simulink model "motor"  (Simulink 8.6)
settings: Solver=FixedStepDiscrete  StartTime=0.0  StopTime=inf  FixedStep=0.002  RelTol=1e-3
PostLoadFcn:
  | ,try, rti_mdl_postloadfcn(bdroot, 'UpdateModel', 160, 'rti1104'); catch, disp(lasterr); end,
undefined symbols (not defined in the file): DiscIntNeverNeededParam
libraries: simulink x3
(part 1 of 3)
CloseFcn:
  | rtwprivate ssgencode ModelCloseRequest two_pisition
settings Model: Creator=Eason  LastModifiedBy=Administrator
settings DataIOCC: SaveFormat=Structure
settings OptimizationCC: BlockReduction=off  OptimizeBlockIOStorage=off  BufferReuse=off  GlobalBufferReuse=off  ExpressionFolding=off  LocalBlockOutputs=off  InitFltsAndDblsToZero=on  OptimizeModelRefInitCode=on  LifeSpan=Inf
settings DebuggingCC: SaveWithParameterizedLinksMsg=none  SignalResolutionControl=TryResolveAllWithWarning  MultiTaskDSMMsg=warning  MultiTaskCondExecSysMsg=none  FcnCallInpInsideContextMsg=UseLocalSettings
settings HardwareCC: ProdLargestAtomicInteger=Long  ProdLargestAtomicFloat=Double  ProdEndianess=LittleEndian  ProdHWDeviceType=ARM Compatible->ARM Cortex  TargetIntDivRoundTo=Zero  TargetEndianess=BigEndian
settings SFSimCC: SimParseCustomCode=off
settings RTWCC: SystemTargetFile=ert.tlc  TemplateMakefile=ert_default_tmf  Description=Embedded Coder  GenerateReport=on  IncludeHyperlinkInReport=on  LaunchReport=on  GenerateTraceInfo=on  GenerateTraceReport=on  GenerateTraceReportSl=on  GenerateTraceReportSf=on  GenerateTraceReportEml=on
settings CodeAppCC: IgnoreCustomStorageClasses=off  CustomSymbolStrType=$N$R$M  InternalIdentifier=Classic
settings ERTTargetCC: MultiwordLength=2048  GenerateSampleERTMain=on  SupportNonFinite=off  SupportComplex=off  ERTCustomFileTemplate=example_file_process.tlc  ConvertIfToSwitch=off  SuppressUnreachableDefaultCases=off
settings ConfigComp: CovSFcnEnable=off

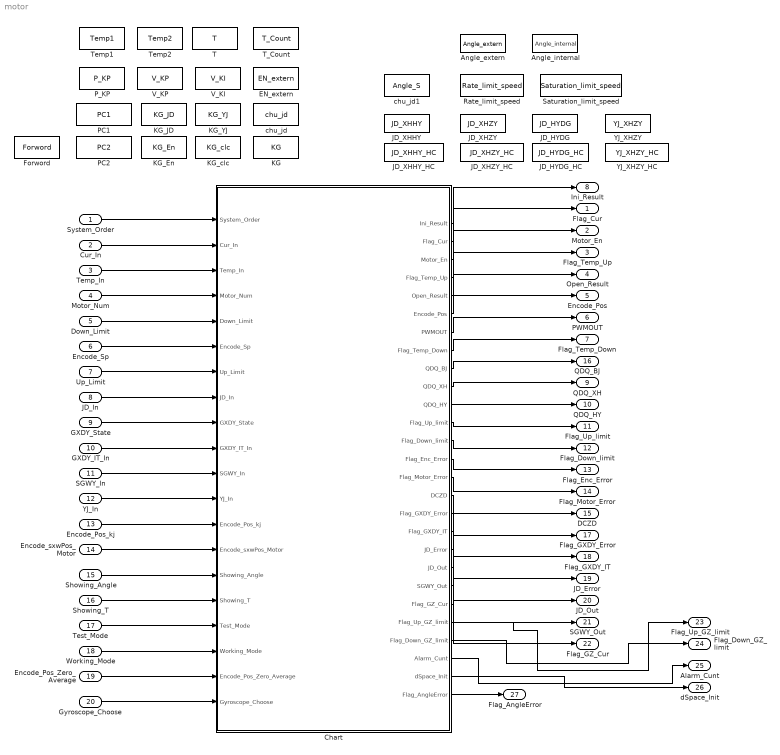
== system motor ==
  System_Order : Inport
  Cur_In : Inport  Port=2  OutDataTypeStr=uint32
  Temp_In : Inport  Port=3  OutDataTypeStr=uint32
  Motor_Num : Inport  Port=4  OutDataTypeStr=uint8
  Down_Limit : Inport  Port=5  OutDataTypeStr=uint8
  Encode_Sp : Inport  Port=6  OutDataTypeStr=int32
  Up_Limit : Inport  Port=7  OutDataTypeStr=uint8
  JD_In : Inport  Port=8  OutDataTypeStr=int32
  GXDY_State : Inport  Port=9  OutDataTypeStr=boolean
  GXDY_IT_In : Inport  Port=10  OutDataTypeStr=uint8
  SGWY_In : Inport  Port=11  OutDataTypeStr=int32
  YJ_In : Inport  Port=12  OutDataTypeStr=int32
  Encode_Pos_kj : Inport  Port=13  OutDataTypeStr=int32
  Encode_sxwPos_Motor : Inport  Port=14  OutDataTypeStr=int32
  Showing_Angle : Inport  Port=15  OutDataTypeStr=int32
  Showing_T : Inport  Port=16  OutDataTypeStr=int32
  Test_Mode : Inport  Port=17  OutDataTypeStr=int32
  Working_Mode : Inport  Port=18  OutDataTypeStr=int32
  Encode_Pos_Zero_Average : Inport  Port=19  OutDataTypeStr=int32
  Gyroscope_Choose : Inport  Port=20  OutDataTypeStr=uint8
  Angle_extern : DataStoreMemory  DataStoreName=Angle_extern  ReadBeforeWriteMsg=warning  WriteAfterWriteMsg=warning  WriteAfterReadMsg=warning  OutDataTypeStr=double
  Angle_internal : DataStoreMemory  DataStoreName=Angle_internal  ReadBeforeWriteMsg=warning  WriteAfterWriteMsg=warning  WriteAfterReadMsg=warning  OutDataTypeStr=double
  Chart : Stateflow chart  TreatAsAtomicUnit=on
  EN_extern : DataStoreMemory  DataStoreName=EN_extern  ReadBeforeWriteMsg=warning  WriteAfterWriteMsg=warning  WriteAfterReadMsg=warning  OutDataTypeStr=uint8
  Forword : DataStoreMemory  DataStoreName=Forword  ReadBeforeWriteMsg=warning  WriteAfterWriteMsg=warning  WriteAfterReadMsg=warning  InitialValue=1  OutDataTypeStr=uint8
  JD_HYDG : DataStoreMemory  DataStoreName=JD_HYDG  ReadBeforeWriteMsg=warning  WriteAfterWriteMsg=warning  WriteAfterReadMsg=warning  OutDataTypeStr=int32
  JD_HYDG_HC : DataStoreMemory  DataStoreName=JD_HYDG_HC  ReadBeforeWriteMsg=warning  WriteAfterWriteMsg=warning  WriteAfterReadMsg=warning  OutDataTypeStr=int32
  JD_XHHY : DataStoreMemory  DataStoreName=JD_XHHY  ReadBeforeWriteMsg=warning  WriteAfterWriteMsg=warning  WriteAfterReadMsg=warning  OutDataTypeStr=int32
  JD_XHHY_HC : DataStoreMemory  DataStoreName=JD_XHHY_HC  ReadBeforeWriteMsg=warning  WriteAfterWriteMsg=warning  WriteAfterReadMsg=warning  OutDataTypeStr=int32
  JD_XHZY : DataStoreMemory  DataStoreName=JD_XHZY  ReadBeforeWriteMsg=warning  WriteAfterWriteMsg=warning  WriteAfterReadMsg=warning  OutDataTypeStr=int32
  JD_XHZY_HC : DataStoreMemory  DataStoreName=JD_XHZY_HC  ReadBeforeWriteMsg=warning  WriteAfterWriteMsg=warning  WriteAfterReadMsg=warning  OutDataTypeStr=int32
  KG : DataStoreMemory  DataStoreName=KG  ReadBeforeWriteMsg=warning  WriteAfterWriteMsg=warning  WriteAfterReadMsg=warning  OutDataTypeStr=uint8
  KG_En : DataStoreMemory  DataStoreName=KG_En  ReadBeforeWriteMsg=warning  WriteAfterWriteMsg=warning  WriteAfterReadMsg=warning  OutDataTypeStr=uint8
  KG_JD : DataStoreMemory  DataStoreName=KG_JD  ReadBeforeWriteMsg=warning  WriteAfterWriteMsg=warning  WriteAfterReadMsg=warning  OutDataTypeStr=uint8
  KG_YJ : DataStoreMemory  DataStoreName=KG_YJ  ReadBeforeWriteMsg=warning  WriteAfterWriteMsg=warning  WriteAfterReadMsg=warning  OutDataTypeStr=uint8
  KG_clc : DataStoreMemory  DataStoreName=KG_clc  ReadBeforeWriteMsg=warning  WriteAfterWriteMsg=warning  WriteAfterReadMsg=warning  OutDataTypeStr=uint8
  PC1 : DataStoreMemory  DataStoreName=PC1  ReadBeforeWriteMsg=warning  WriteAfterWriteMsg=warning  WriteAfterReadMsg=warning  OutDataTypeStr=boolean
  PC2 : DataStoreMemory  DataStoreName=PC2  ReadBeforeWriteMsg=warning  WriteAfterWriteMsg=warning  WriteAfterReadMsg=warning  OutDataTypeStr=boolean
  P_KP : DataStoreMemory  DataStoreName=P_KP  ReadBeforeWriteMsg=warning  WriteAfterWriteMsg=warning  WriteAfterReadMsg=warning  InitialValue=330  OutDataTypeStr=double
  Rate_limit_speed : DataStoreMemory  DataStoreName=Rate_limit_speed  ReadBeforeWriteMsg=warning  WriteAfterWriteMsg=warning  WriteAfterReadMsg=warning  InitialValue=50000  OutDataTypeStr=double
  Saturation_limit_speed : DataStoreMemory  DataStoreName=Saturation_limit_speed  ReadBeforeWriteMsg=warning  WriteAfterWriteMsg=warning  WriteAfterReadMsg=warning  InitialValue=16000  OutDataTypeStr=double
  T : DataStoreMemory  DataStoreName=T  ReadBeforeWriteMsg=warning  WriteAfterWriteMsg=warning  WriteAfterReadMsg=warning  OutDataTypeStr=double
  T_Count : DataStoreMemory  DataStoreName=T_Count  ReadBeforeWriteMsg=warning  WriteAfterWriteMsg=warning  WriteAfterReadMsg=warning  OutDataTypeStr=double
  Temp1 : DataStoreMemory  DataStoreName=Temp1  ReadBeforeWriteMsg=warning  WriteAfterWriteMsg=warning  WriteAfterReadMsg=warning  OutDataTypeStr=double
  Temp2 : DataStoreMemory  DataStoreName=Temp2  ReadBeforeWriteMsg=warning  WriteAfterWriteMsg=warning  WriteAfterReadMsg=warning  OutDataTypeStr=double
  V_KI : DataStoreMemory  DataStoreName=V_KI  ReadBeforeWriteMsg=warning  WriteAfterWriteMsg=warning  WriteAfterReadMsg=warning  InitialValue=10  OutDataTypeStr=double
  V_KP : DataStoreMemory  DataStoreName=V_KP  ReadBeforeWriteMsg=warning  WriteAfterWriteMsg=warning  WriteAfterReadMsg=warning  InitialValue=1  OutDataTypeStr=double
  YJ_XHZY : DataStoreMemory  DataStoreName=YJ_XHZY  ReadBeforeWriteMsg=warning  WriteAfterWriteMsg=warning  WriteAfterReadMsg=warning  OutDataTypeStr=int32
  YJ_XHZY_HC : DataStoreMemory  DataStoreName=YJ_XHZY_HC  ReadBeforeWriteMsg=warning  WriteAfterWriteMsg=warning  WriteAfterReadMsg=warning  OutDataTypeStr=int32
  chu_jd : DataStoreMemory  DataStoreName=chu_jd  ReadBeforeWriteMsg=warning  WriteAfterWriteMsg=warning  WriteAfterReadMsg=warning  OutDataTypeStr=double
  chu_jd1 : DataStoreMemory  DataStoreName=Angle_S  ReadBeforeWriteMsg=warning  WriteAfterWriteMsg=warning  WriteAfterReadMsg=warning  OutDataTypeStr=double
  Flag_Cur : Outport  OutDataTypeStr=uint8
  Motor_En : Outport  Port=2  OutDataTypeStr=boolean
  Flag_Temp_Up : Outport  Port=3  OutDataTypeStr=uint8
  Open_Result : Outport  Port=4  OutDataTypeStr=uint8
  Encode_Pos : Outport  Port=5  OutDataTypeStr=int32
  PWMOUT : Outport  Port=6  OutDataTypeStr=uint16
  Flag_Temp_Down : Outport  Port=7  OutDataTypeStr=uint8
  Ini_Result : Outport  Port=8  OutDataTypeStr=uint8
  QDQ_XH : Outport  Port=9  OutDataTypeStr=boolean
  QDQ_HY : Outport  Port=10  OutDataTypeStr=boolean
  Flag_Up_limit : Outport  Port=11  OutDataTypeStr=uint8
  Flag_Down_limit : Outport  Port=12  OutDataTypeStr=uint8
  Flag_Enc_Error : Outport  Port=13  OutDataTypeStr=uint8
  Flag_Motor_Error : Outport  Port=14  OutDataTypeStr=uint8
  DCZD : Outport  Port=15  OutDataTypeStr=boolean
  QDQ_BJ : Outport  Port=16  OutDataTypeStr=uint8
  Flag_GXDY_Error : Outport  Port=17  OutDataTypeStr=uint8
  Flag_GXDY_IT : Outport  Port=18  OutDataTypeStr=uint8
  JD_Error : Outport  Port=19  OutDataTypeStr=int32
  JD_Out : Outport  Port=20  OutDataTypeStr=int32
  SGWY_Out : Outport  Port=21  OutDataTypeStr=int32
  Flag_GZ_Cur : Outport  Port=22  OutDataTypeStr=uint8
  Flag_Up_GZ_limit : Outport  Port=23  OutDataTypeStr=uint8
  Flag_Down_GZ_limit : Outport  Port=24  OutDataTypeStr=uint8
  Alarm_Cunt : Outport  Port=25  OutDataTypeStr=uint8
  dSpace_Init : Outport  Port=26  OutDataTypeStr=uint8
  Flag_AngleError : Outport  Port=27  OutDataTypeStr=uint8
  wires:
  Chart/2(Flag_Cur) -> Flag_Cur/1
  Chart/3(Motor_En) -> Motor_En/1
  Temp_In/1 -> Chart/3(Temp_In)
  Chart/4(Flag_Temp_Up) -> Flag_Temp_Up/1
  Chart/5(Open_Result) -> Open_Result/1
  Motor_Num/1 -> Chart/4(Motor_Num)
  Chart/6(Encode_Pos) -> Encode_Pos/1
  Chart/7(PWMOUT) -> PWMOUT/1
  Chart/8(Flag_Temp_Down) -> Flag_Temp_Down/1
  Chart/1(Ini_Result) -> Ini_Result/1
  Chart/10(QDQ_XH) -> QDQ_XH/1
  Chart/11(QDQ_HY) -> QDQ_HY/1
  Cur_In/1 -> Chart/2(Cur_In)
  System_Order/1 -> Chart/1(System_Order)
  Chart/12(Flag_Up_limit) -> Flag_Up_limit/1
  Chart/13(Flag_Down_limit) -> Flag_Down_limit/1
  Chart/14(Flag_Enc_Error) -> Flag_Enc_Error/1
  Chart/15(Flag_Motor_Error) -> Flag_Motor_Error/1
  Chart/16(DCZD) -> DCZD/1
  Down_Limit/1 -> Chart/5(Down_Limit)
  Encode_Sp/1 -> Chart/6(Encode_Sp)
  Chart/9(QDQ_BJ) -> QDQ_BJ/1
  JD_In/1 -> Chart/8(JD_In)
  Chart/17(Flag_GXDY_Error) -> Flag_GXDY_Error/1
  GXDY_State/1 -> Chart/9(GXDY_State)
  GXDY_IT_In/1 -> Chart/10(GXDY_IT_In)
  Chart/18(Flag_GXDY_IT) -> Flag_GXDY_IT/1
  SGWY_In/1 -> Chart/11(SGWY_In)
  YJ_In/1 -> Chart/12(YJ_In)
  Chart/19(JD_Error) -> JD_Error/1
  Chart/20(JD_Out) -> JD_Out/1
  Chart/21(SGWY_Out) -> SGWY_Out/1
  Chart/22(Flag_GZ_Cur) -> Flag_GZ_Cur/1
  Chart/23(Flag_Up_GZ_limit) -> Flag_Up_GZ_limit/1
  Chart/24(Flag_Down_GZ_limit) -> Flag_Down_GZ_limit/1
  Chart/25(Alarm_Cunt) -> Alarm_Cunt/1
  Encode_Pos_kj/1 -> Chart/13(Encode_Pos_kj)
  Encode_sxwPos_Motor/1 -> Chart/14(Encode_sxwPos_Motor)
  Up_Limit/1 -> Chart/7(Up_Limit)
  Showing_Angle/1 -> Chart/15(Showing_Angle)
  Showing_T/1 -> Chart/16(Showing_T)
  Test_Mode/1 -> Chart/17(Test_Mode)
  Working_Mode/1 -> Chart/18(Working_Mode)
  Encode_Pos_Zero_Average/1 -> Chart/19(Encode_Pos_Zero_Average)
  Gyroscope_Choose/1 -> Chart/20(Gyroscope_Choose)
  Chart/26(dSpace_Init) -> dSpace_Init/1
  Chart/27(Flag_AngleError) -> Flag_AngleError/1

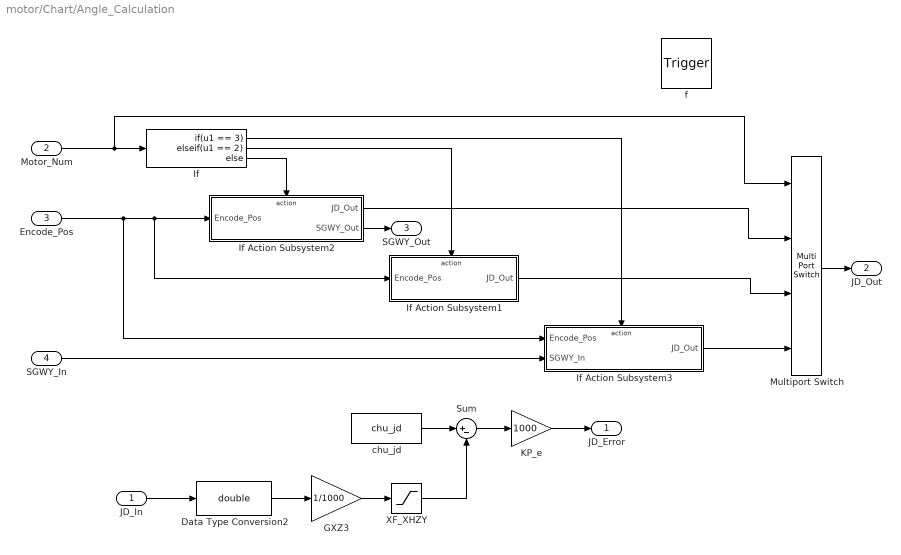
== system motor/Chart/Angle_Calculation ==
  JD_In : Inport  OutDataTypeStr=int32  PortDimensions=1
  Motor_Num : Inport  Port=2  OutDataTypeStr=uint8  PortDimensions=1
  Encode_Pos : Inport  Port=3  OutDataTypeStr=uint8  PortDimensions=1
  SGWY_In : Inport  Port=4  OutDataTypeStr=uint8  PortDimensions=1
  f : TriggerPort  TriggerType=function-call
      settings: CopyFcn=Stateflow.SLINSF.SimulinkMan.removeBlockPreDeleteFcn  PreDeleteFcn=Stateflow.SLINSF.SimulinkMan.unsafePredeleteFcn
  Data Type Conversion2 : DataTypeConversion  OutDataTypeStr=double
  GXZ3 : Gain  Gain=1/1000
  If : If  IfExpression=u1 == 3  ElseIfExpressions=u1 == 2
  If Action Subsystem1 : Subsystem  TreatAsAtomicUnit=on
  If Action Subsystem2 : Subsystem  TreatAsAtomicUnit=on
  If Action Subsystem3 : Subsystem  TreatAsAtomicUnit=on
  KP_e : Gain  Gain=1000
  Multiport Switch : MultiPortSwitch
  Sum : Sum  Inputs=|+-
  XF_XHZY : Saturate  UpperLimit=15  LowerLimit=-15
  chu_jd : DataStoreRead  DataStoreName=chu_jd
  JD_Error : Outport
  JD_Out : Outport  Port=2
  SGWY_Out : Outport  Port=3
  wires:
  GXZ3/1 -> XF_XHZY/1
  XF_XHZY/1 -> Sum/2
  Data Type Conversion2/1 -> GXZ3/1
  If/1 -> If Action Subsystem3/Action
  If/2 -> If Action Subsystem1/Action
  If/3 -> If Action Subsystem2/Action
  Motor_Num/1 -> Multiport Switch/1, If/1
  JD_In/1 -> Data Type Conversion2/1
  Sum/1 -> KP_e/1
  KP_e/1 -> JD_Error/1
  chu_jd/1 -> Sum/1
  Encode_Pos/1 -> If Action Subsystem3/1(Encode_Pos), If Action Subsystem1/1(Encode_Pos), If Action Subsystem2/1(Encode_Pos)
  SGWY_In/1 -> If Action Subsystem3/2(SGWY_In)
  If Action Subsystem2/2(SGWY_Out) -> SGWY_Out/1
  If Action Subsystem3/1(JD_Out) -> Multiport Switch/4
  If Action Subsystem1/1(JD_Out) -> Multiport Switch/3
  If Action Subsystem2/1(JD_Out) -> Multiport Switch/2
  Multiport Switch/1 -> JD_Out/1

== system motor/Chart/Angle_Calculation_HY ==
  Encode_Pos : Inport  OutDataTypeStr=int32  PortDimensions=1
  f : TriggerPort  TriggerType=function-call
      settings: CopyFcn=Stateflow.SLINSF.SimulinkMan.removeBlockPreDeleteFcn  PreDeleteFcn=Stateflow.SLINSF.SimulinkMan.unsafePredeleteFcn
  Data Type Conversion1 : DataTypeConversion  OutDataTypeStr=double
  GHDG5 : Gain  Gain=360/65536
  fs_plat : Subsystem
  Angle_Calculation : Outport
  wires:
  Encode_Pos/1 -> Data Type Conversion1/1
  Data Type Conversion1/1 -> GHDG5/1
  GHDG5/1 -> fs_plat/1(In1)
  fs_plat/1(Out1) -> Angle_Calculation/1

== system motor/Chart/Angle_Calculation_XH ==
  Encode_Pos : Inport  OutDataTypeStr=int32  PortDimensions=1
  f : TriggerPort  TriggerType=function-call
      settings: CopyFcn=Stateflow.SLINSF.SimulinkMan.removeBlockPreDeleteFcn  PreDeleteFcn=Stateflow.SLINSF.SimulinkMan.unsafePredeleteFcn
  Data Type Conversion2 : DataTypeConversion  OutDataTypeStr=double
  GXZ1 : Gain  Gain=1/322
  GXZ6 : Gain  Gain=360/65536
  Angle_Calculation : Outport
  wires:
  Encode_Pos/1 -> Data Type Conversion2/1
  GXZ6/1 -> GXZ1/1
  Data Type Conversion2/1 -> GXZ6/1
  GXZ1/1 -> Angle_Calculation/1

== system motor/Chart/BJ ==
  x : Inport  OutDataTypeStr=uint8
  y : Inport  Port=2
  f : TriggerPort  TriggerType=function-call
      settings: CopyFcn=Stateflow.SLINSF.SimulinkMan.removeBlockPreDeleteFcn  PreDeleteFcn=Stateflow.SLINSF.SimulinkMan.unsafePredeleteFcn
  Data Store Read : DataStoreRead  DataStoreName=PC2
  Data Store Read1 : DataStoreRead  DataStoreName=PC1
  If Action Subsystem : Subsystem  TreatAsAtomicUnit=on
  If Action Subsystem1 : Subsystem  TreatAsAtomicUnit=on
  If Action Subsystem2 : Subsystem  TreatAsAtomicUnit=on
  Switch Case : SwitchCase  CaseConditions={1 2 3}  ShowDefaultCase=off
  Out1 : Outport  OutDataTypeStr=boolean
  Out2 : Outport  Port=2  OutDataTypeStr=boolean
  wires:
  Switch Case/1 -> If Action Subsystem/Action
  Switch Case/2 -> If Action Subsystem1/Action
  Switch Case/3 -> If Action Subsystem2/Action
  y/1 -> If Action Subsystem2/1(In1), If Action Subsystem1/1(In1), If Action Subsystem/1(In1)
  x/1 -> Switch Case/1
  Data Store Read1/1 -> Out1/1
  Data Store Read/1 -> Out2/1

== system motor/Chart/COM_Error ==
  In : Inport
  f : TriggerPort  TriggerType=function-call
      settings: CopyFcn=Stateflow.SLINSF.SimulinkMan.removeBlockPreDeleteFcn  PreDeleteFcn=Stateflow.SLINSF.SimulinkMan.unsafePredeleteFcn
  Abs : Abs
  Add : Sum  Inputs=+-
  Unit Delay : UnitDelay  SampleTime=-1
  Out : Outport
  wires:
  In/1 -> Unit Delay/1, Add/1
  Unit Delay/1 -> Add/2
  Add/1 -> Abs/1
  Abs/1 -> Out/1

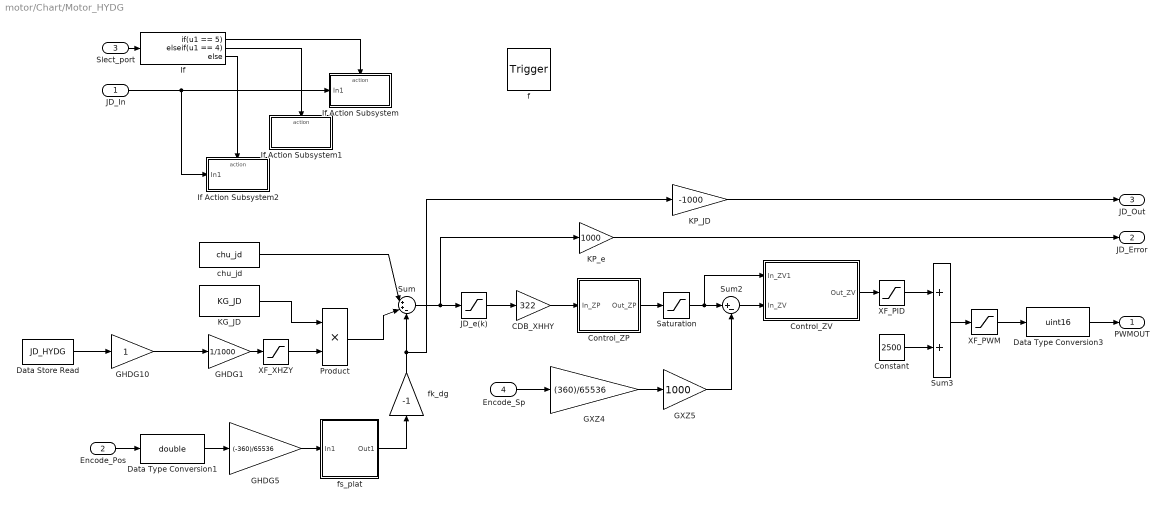
== system motor/Chart/Motor_HYDG ==
  JD_In : Inport  OutDataTypeStr=int32  PortDimensions=1
  Encode_Pos : Inport  Port=2  OutDataTypeStr=int32  PortDimensions=1
  Slect_port : Inport  Port=3  OutDataTypeStr=uint8  PortDimensions=1
  Encode_Sp : Inport  Port=4  OutDataTypeStr=int32  PortDimensions=1
  f : TriggerPort  TriggerType=function-call
      settings: CopyFcn=Stateflow.SLINSF.SimulinkMan.removeBlockPreDeleteFcn  PreDeleteFcn=Stateflow.SLINSF.SimulinkMan.unsafePredeleteFcn
  CDB_XHHY : Gain  Gain=322
  Constant : Constant  Value=2500
  Control_ZP : Subsystem
  Control_ZV : Subsystem
  Data Store Read : DataStoreRead  DataStoreName=JD_HYDG
  Data Type Conversion1 : DataTypeConversion  OutDataTypeStr=double
  Data Type Conversion3 : DataTypeConversion  OutDataTypeStr=uint16
  GHDG1 : Gain  Gain=1/1000
  GHDG10 : Gain
  GHDG5 : Gain  Gain=(-360)/65536
  GXZ4 : Gain  Gain=(360)/65536
  GXZ5 : Gain  Gain=1000
  If : If  IfExpression=u1 == 5  ElseIfExpressions=u1 == 4
  If Action Subsystem : Subsystem  TreatAsAtomicUnit=on
  If Action Subsystem1 : Subsystem  TreatAsAtomicUnit=on
  If Action Subsystem2 : Subsystem  TreatAsAtomicUnit=on
  JD_e(k) : Saturate  UpperLimit=15  LowerLimit=-15
  KG_JD : DataStoreRead  DataStoreName=KG_JD
  KP_JD : Gain  Gain=-1000
  KP_e : Gain  Gain=1000
  Product : Product  OutDataTypeStr=double
  Saturation : Saturate  UpperLimit=8000  LowerLimit=-8000
  Sum : Sum  Inputs=|++-
  Sum2 : Sum  Inputs=|+-
  Sum3 : Sum
  XF_PID : Saturate  UpperLimit=2500  LowerLimit=-2500
  XF_PWM : Saturate  UpperLimit=4000  LowerLimit=1000
  XF_XHZY : Saturate  UpperLimit=15  LowerLimit=-15
  chu_jd : DataStoreRead  DataStoreName=chu_jd
  fk_dg : Gain  Gain=-1
  fs_plat : Subsystem
  PWMOUT : Outport
  JD_Error : Outport  Port=2
  JD_Out : Outport  Port=3
  wires:
  Product/1 -> Sum/2
  Control_ZV/1(Out_ZV) -> XF_PID/1
  XF_PID/1 -> Sum3/1
  Constant/1 -> Sum3/2
  Sum3/1 -> XF_PWM/1
  XF_PWM/1 -> Data Type Conversion3/1
  GHDG10/1 -> GHDG1/1
  GHDG1/1 -> XF_XHZY/1
  KG_JD/1 -> Product/1
  Encode_Pos/1 -> Data Type Conversion1/1
  Data Type Conversion3/1 -> PWMOUT/1
  KP_JD/1 -> JD_Out/1
  KP_e/1 -> JD_Error/1
  Data Store Read/1 -> GHDG10/1
  JD_In/1 -> If Action Subsystem2/1(In1), If Action Subsystem/1(In1)
  If/1 -> If Action Subsystem/Action
  If/2 -> If Action Subsystem1/Action
  If/3 -> If Action Subsystem2/Action
  Slect_port/1 -> If/1
  Data Type Conversion1/1 -> GHDG5/1
  GXZ4/1 -> GXZ5/1
  Encode_Sp/1 -> GXZ4/1
  XF_XHZY/1 -> Product/2
  CDB_XHHY/1 -> Control_ZP/1(In_ZP)
  Control_ZP/1(Out_ZP) -> Saturation/1
  Sum2/1 -> Control_ZV/2(In_ZV)
  Sum/1 -> KP_e/1, JD_e(k)/1
  Saturation/1 -> Sum2/1, Control_ZV/1(In_ZV1)
  JD_e(k)/1 -> CDB_XHHY/1
  GXZ5/1 -> Sum2/2
  fk_dg/1 -> KP_JD/1, Sum/3
  chu_jd/1 -> Sum/1
  GHDG5/1 -> fs_plat/1(In1)
  fs_plat/1(Out1) -> fk_dg/1

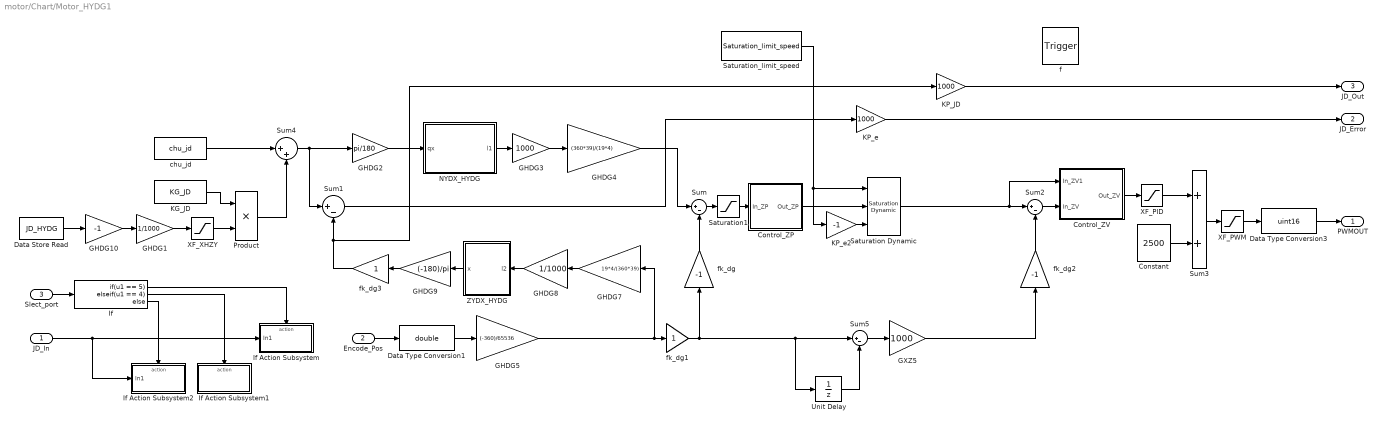
== system motor/Chart/Motor_HYDG1 ==
  JD_In : Inport  OutDataTypeStr=int32  PortDimensions=1
  Encode_Pos : Inport  Port=2  OutDataTypeStr=int32  PortDimensions=1
  Slect_port : Inport  Port=3  OutDataTypeStr=uint8  PortDimensions=1
  f : TriggerPort  TriggerType=function-call
      settings: CopyFcn=Stateflow.SLINSF.SimulinkMan.removeBlockPreDeleteFcn  PreDeleteFcn=Stateflow.SLINSF.SimulinkMan.unsafePredeleteFcn
  Constant : Constant  Value=2500
  Control_ZP : Subsystem
  Control_ZV : Subsystem
  Data Store Read : DataStoreRead  DataStoreName=JD_HYDG
  Data Type Conversion1 : DataTypeConversion  OutDataTypeStr=double
  Data Type Conversion3 : DataTypeConversion  OutDataTypeStr=uint16
  GHDG1 : Gain  Gain=1/1000
  GHDG10 : Gain  Gain=-1
  GHDG2 : Gain  Gain=pi/180
  GHDG3 : Gain  Gain=1000
  GHDG4 : Gain  Gain=(360*39)/(19*4)
  GHDG5 : Gain  Gain=(-360)/65536
  GHDG7 : Gain  Gain=19*4/(360*39)
  GHDG8 : Gain  Gain=1/1000
  GHDG9 : Gain  Gain=(-180)/pi
  GXZ5 : Gain  Gain=1000
  If : If  IfExpression=u1 == 5  ElseIfExpressions=u1 == 4
  If Action Subsystem : Subsystem  TreatAsAtomicUnit=on
  If Action Subsystem1 : Subsystem  TreatAsAtomicUnit=on
  If Action Subsystem2 : Subsystem  TreatAsAtomicUnit=on
  KG_JD : DataStoreRead  DataStoreName=KG_JD
  KP_JD : Gain  Gain=1000
  KP_e : Gain  Gain=1000
  KP_e2 : Gain  Gain=-1
  NYDX_HYDG : Subsystem
  Product : Product  OutDataTypeStr=double
  Saturation Dynamic : simulink/Discontinuities/Saturation Dynamic  OutMin=[]  OutMax=[]  OutDataTypeStr=Inherit: Same as second input  OutDataType=fixdt(1, 16)  OutScaling=2^-10  DoSatur=off
  Saturation1 : Saturate  UpperLimit=200  LowerLimit=-200
  Saturation_limit_speed : DataStoreRead  DataStoreName=Saturation_limit_speed
  Sum{,1..2,5} (4 alike) : Sum  Inputs=|+-
  Sum3 : Sum
  Sum4 : Sum  Inputs=|++
  Unit Delay : UnitDelay  SampleTime=-1
  XF_PID : Saturate  UpperLimit=2500  LowerLimit=-2500
  XF_PWM : Saturate  UpperLimit=4900  LowerLimit=100
  XF_XHZY : Saturate  UpperLimit=20  LowerLimit=-20
  ZYDX_HYDG : Subsystem
  chu_jd : DataStoreRead  DataStoreName=chu_jd
  fk_dg : Gain  Gain=-1
  fk_dg1 : Gain
  fk_dg2 : Gain  Gain=-1
  fk_dg3 : Gain
  PWMOUT : Outport
  JD_Error : Outport  Port=2
  JD_Out : Outport  Port=3
  wires:
  GHDG4/1 -> Sum/1
  Control_ZV/1(Out_ZV) -> XF_PID/1
  XF_PID/1 -> Sum3/1
  Constant/1 -> Sum3/2
  Sum3/1 -> XF_PWM/1
  XF_PWM/1 -> Data Type Conversion3/1
  GHDG10/1 -> GHDG1/1
  GHDG1/1 -> XF_XHZY/1
  KG_JD/1 -> Product/1
  Encode_Pos/1 -> Data Type Conversion1/1
  Data Type Conversion3/1 -> PWMOUT/1
  KP_JD/1 -> JD_Out/1
  KP_e/1 -> JD_Error/1
  Data Store Read/1 -> GHDG10/1
  JD_In/1 -> If Action Subsystem2/1(In1), If Action Subsystem/1(In1)
  If/1 -> If Action Subsystem/Action
  If/2 -> If Action Subsystem1/Action
  If/3 -> If Action Subsystem2/Action
  Slect_port/1 -> If/1
  Data Type Conversion1/1 -> GHDG5/1
  XF_XHZY/1 -> Product/2
  Sum/1 -> Saturation1/1
  Control_ZP/1(Out_ZP) -> Saturation Dynamic/2
  Sum2/1 -> Control_ZV/2(In_ZV)
  GXZ5/1 -> fk_dg2/1
  fk_dg/1 -> Sum/2
  GHDG2/1 -> NYDX_HYDG/1(qx)
  NYDX_HYDG/1(l1) -> GHDG3/1
  GHDG3/1 -> GHDG4/1
  Product/1 -> Sum4/2
  GHDG5/1 -> fk_dg1/1, GHDG7/1
  GHDG7/1 -> GHDG8/1
  GHDG8/1 -> ZYDX_HYDG/1(l2)
  ZYDX_HYDG/1(x) -> GHDG9/1
  Sum1/1 -> KP_e/1
  GHDG9/1 -> fk_dg3/1
  fk_dg3/1 -> Sum1/2, KP_JD/1
  Sum5/1 -> GXZ5/1
  Sum4/1 -> Sum1/1, GHDG2/1
  chu_jd/1 -> Sum4/1
  Unit Delay/1 -> Sum5/2
  fk_dg1/1 -> Unit Delay/1, Sum5/1, fk_dg/1
  fk_dg2/1 -> Sum2/2
  Saturation1/1 -> Control_ZP/1(In_ZP)
  Saturation Dynamic/1 -> Sum2/1, Control_ZV/1(In_ZV1)
  Saturation_limit_speed/1 -> KP_e2/1, Saturation Dynamic/1
  KP_e2/1 -> Saturation Dynamic/3

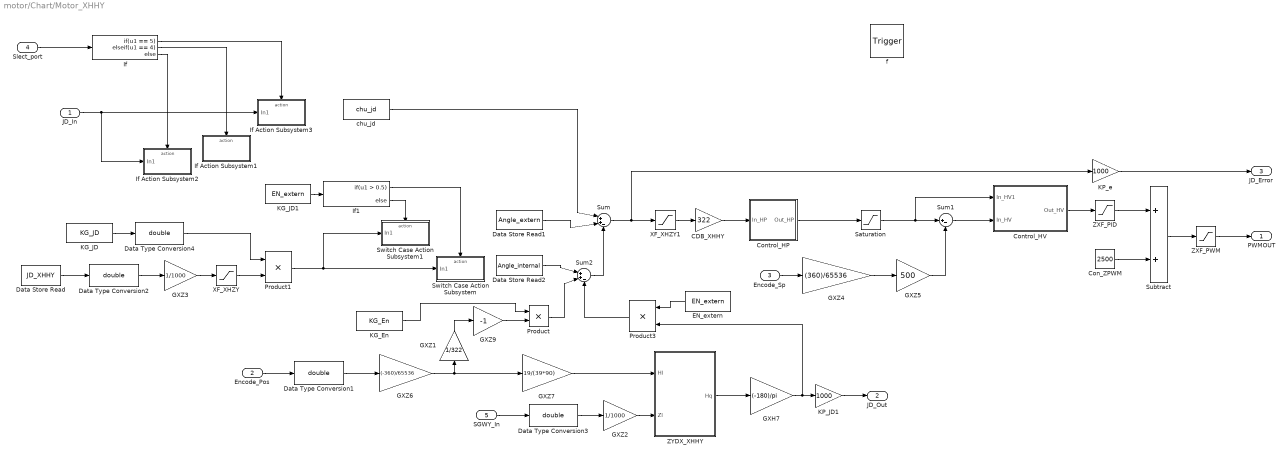
== system motor/Chart/Motor_XHHY ==
  JD_In : Inport  OutDataTypeStr=int32  PortDimensions=1
  Encode_Pos : Inport  Port=2  OutDataTypeStr=int32  PortDimensions=1
  Encode_Sp : Inport  Port=3  OutDataTypeStr=int32  PortDimensions=1
  Slect_port : Inport  Port=4  OutDataTypeStr=uint8  PortDimensions=1
  SGWY_In : Inport  Port=5  OutDataTypeStr=int32  PortDimensions=1
  f : TriggerPort  TriggerType=function-call
      settings: CopyFcn=Stateflow.SLINSF.SimulinkMan.removeBlockPreDeleteFcn  PreDeleteFcn=Stateflow.SLINSF.SimulinkMan.unsafePredeleteFcn
  CDB_XHHY : Gain  Gain=322
  Con_ZPWM : Constant  Value=2500
  Control_HP : Subsystem
  Control_HV : Subsystem
  Data Store Read : DataStoreRead  DataStoreName=JD_XHHY
  Data Store Read1 : DataStoreRead  DataStoreName=Angle_extern
  Data Store Read2 : DataStoreRead  DataStoreName=Angle_internal
  Data Type Conversion{1..4} (4 alike) : DataTypeConversion  OutDataTypeStr=double
  EN_extern : DataStoreRead  DataStoreName=EN_extern
  GXH7 : Gain  Gain=(-180)/pi
  GXZ1 : Gain  Gain=1/322
  GXZ2 : Gain  Gain=1/1000
  GXZ3 : Gain  Gain=1/1000
  GXZ4 : Gain  Gain=(360)/65536
  GXZ5 : Gain  Gain=500
  GXZ6 : Gain  Gain=(-360)/65536
  GXZ7 : Gain  Gain=19/(39*90)
  GXZ9 : Gain  Gain=-1
  If : If  IfExpression=u1 == 5  ElseIfExpressions=u1 == 4
  If Action Subsystem1 : Subsystem  TreatAsAtomicUnit=on
  If Action Subsystem2 : Subsystem  TreatAsAtomicUnit=on
  If Action Subsystem3 : Subsystem  TreatAsAtomicUnit=on
  If1 : If  IfExpression=u1 > 0.5
  KG_En : DataStoreRead  DataStoreName=KG_En
  KG_JD : DataStoreRead  DataStoreName=KG_JD
  KG_JD1 : DataStoreRead  DataStoreName=EN_extern
  KP_JD1 : Gain  Gain=1000
  KP_e : Gain  Gain=1000
  Product : Product
  Product1 : Product
  Product3 : Product
  Saturation : Saturate  UpperLimit=6600  LowerLimit=-6600
  Subtract : Sum
  Sum : Sum  Inputs=|++-
  Sum1 : Sum  Inputs=|+-
  Sum2 : Sum  Inputs=|++-
  Switch Case Action Subsystem : Subsystem  TreatAsAtomicUnit=on
  Switch Case Action Subsystem1 : Subsystem  TreatAsAtomicUnit=on
  XF_XHZY : Saturate  UpperLimit=15  LowerLimit=-15
  XF_XHZY1 : Saturate  UpperLimit=15  LowerLimit=-15
  ZXF_PID : Saturate  UpperLimit=2500  LowerLimit=-2500
  ZXF_PWM : Saturate  UpperLimit=4800  LowerLimit=200
  ZYDX_XHHY : Subsystem
  chu_jd : DataStoreRead  DataStoreName=chu_jd
  PWMOUT : Outport
  JD_Out : Outport  Port=2
  JD_Error : Outport  Port=3
  wires:
  CDB_XHHY/1 -> Control_HP/1(In_HP)
  Control_HP/1(Out_HP) -> Saturation/1
  Sum1/1 -> Control_HV/2(In_HV)
  Control_HV/1(Out_HV) -> ZXF_PID/1
  ZXF_PID/1 -> Subtract/1
  Con_ZPWM/1 -> Subtract/2
  Subtract/1 -> ZXF_PWM/1
  ZXF_PWM/1 -> PWMOUT/1
  GXZ5/1 -> Sum1/2
  Encode_Sp/1 -> GXZ4/1
  GXZ4/1 -> GXZ5/1
  Encode_Pos/1 -> Data Type Conversion1/1
  GXZ6/1 -> GXZ7/1, GXZ1/1
  GXZ3/1 -> XF_XHZY/1
  Saturation/1 -> Control_HV/1(In_HV1), Sum1/1
  GXZ1/1 -> GXZ9/1
  Product/1 -> Sum2/2
  KG_En/1 -> Product/1
  Data Type Conversion1/1 -> GXZ6/1
  Data Type Conversion2/1 -> GXZ3/1
  JD_In/1 -> If Action Subsystem3/1(In1), If Action Subsystem2/1(In1)
  If/1 -> If Action Subsystem3/Action
  If/2 -> If Action Subsystem1/Action
  If/3 -> If Action Subsystem2/Action
  Slect_port/1 -> If/1
  Data Store Read/1 -> Data Type Conversion2/1
  Sum/1 -> XF_XHZY1/1, KP_e/1
  GXZ9/1 -> Product/2
  KP_e/1 -> JD_Error/1
  ZYDX_XHHY/1(Hq) -> GXH7/1
  GXZ7/1 -> ZYDX_XHHY/1(Hl)
  SGWY_In/1 -> Data Type Conversion3/1
  GXZ2/1 -> ZYDX_XHHY/2(Zl)
  KP_JD1/1 -> JD_Out/1
  Data Type Conversion3/1 -> GXZ2/1
  XF_XHZY1/1 -> CDB_XHHY/1
  XF_XHZY/1 -> Product1/2
  KG_JD/1 -> Data Type Conversion4/1
  Data Type Conversion4/1 -> Product1/1
  chu_jd/1 -> Sum/1
  GXH7/1 -> Product3/2, KP_JD1/1
  Product3/1 -> Sum2/3
  EN_extern/1 -> Product3/1
  Sum2/1 -> Sum/3
  KG_JD1/1 -> If1/1
  If1/1 -> Switch Case Action Subsystem/Action
  Data Store Read1/1 -> Sum/2
  Data Store Read2/1 -> Sum2/1
  Product1/1 -> Switch Case Action Subsystem1/1(In1), Switch Case Action Subsystem/1(In1)
  If1/2 -> Switch Case Action Subsystem1/Action

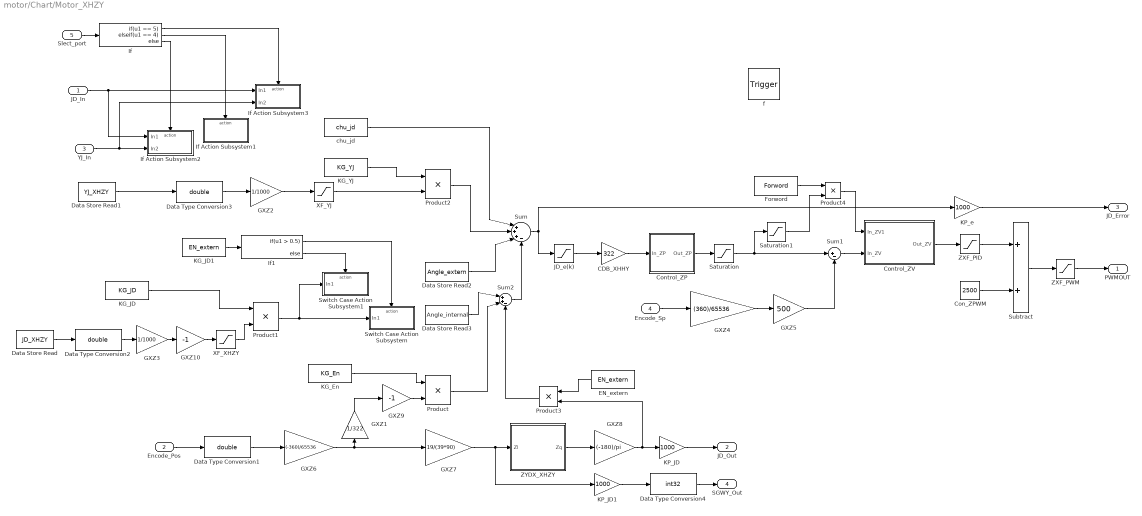
== system motor/Chart/Motor_XHZY ==
  JD_In : Inport  OutDataTypeStr=int32  PortDimensions=1
  Encode_Pos : Inport  Port=2  OutDataTypeStr=int32  PortDimensions=1
  YJ_In : Inport  Port=3  OutDataTypeStr=int32  PortDimensions=1
  Encode_Sp : Inport  Port=4  OutDataTypeStr=int32  PortDimensions=1
  Slect_port : Inport  Port=5  OutDataTypeStr=uint8  PortDimensions=1
  f : TriggerPort  TriggerType=function-call
      settings: CopyFcn=Stateflow.SLINSF.SimulinkMan.removeBlockPreDeleteFcn  PreDeleteFcn=Stateflow.SLINSF.SimulinkMan.unsafePredeleteFcn
  CDB_XHHY : Gain  Gain=322
  Con_ZPWM : Constant  Value=2500
  Control_ZP : Subsystem
  Control_ZV : Subsystem
  Data Store Read : DataStoreRead  DataStoreName=JD_XHZY
  Data Store Read1 : DataStoreRead  DataStoreName=YJ_XHZY
  Data Store Read2 : DataStoreRead  DataStoreName=Angle_extern
  Data Store Read3 : DataStoreRead  DataStoreName=Angle_internal
  Data Type Conversion1 : DataTypeConversion  OutDataTypeStr=double
  Data Type Conversion2 : DataTypeConversion  OutDataTypeStr=double
  Data Type Conversion3 : DataTypeConversion  OutDataTypeStr=double
  Data Type Conversion4 : DataTypeConversion  OutDataTypeStr=int32
  EN_extern : DataStoreRead  DataStoreName=EN_extern
  Forword : DataStoreRead  DataStoreName=Forword
  GXZ1 : Gain  Gain=1/322
  GXZ10 : Gain  Gain=-1
  GXZ2 : Gain  Gain=1/1000
  GXZ3 : Gain  Gain=1/1000
  GXZ4 : Gain  Gain=(360)/65536
  GXZ5 : Gain  Gain=500
  GXZ6 : Gain  Gain=(-360)/65536
  GXZ7 : Gain  Gain=19/(39*90)
  GXZ8 : Gain  Gain=(-180)/pi
  GXZ9 : Gain  Gain=-1
  If : If  IfExpression=u1 == 5  ElseIfExpressions=u1 == 4
  If Action Subsystem1 : Subsystem  TreatAsAtomicUnit=on
  If Action Subsystem2 : Subsystem  TreatAsAtomicUnit=on
  If Action Subsystem3 : Subsystem  TreatAsAtomicUnit=on
  If1 : If  IfExpression=u1 > 0.5
  JD_e(k) : Saturate  UpperLimit=15  LowerLimit=-15
  KG_En : DataStoreRead  DataStoreName=KG_En
  KG_JD : DataStoreRead  DataStoreName=KG_JD
  KG_JD1 : DataStoreRead  DataStoreName=EN_extern
  KG_YJ : DataStoreRead  DataStoreName=KG_YJ
  KP_JD : Gain  Gain=1000
  KP_JD1 : Gain  Gain=1000
  KP_e : Gain  Gain=1000
  Product{,1..4} (5 alike) : Product
  Saturation : Saturate  UpperLimit=8000  LowerLimit=-8000
  Saturation1 : Saturate  UpperLimit=3000  LowerLimit=-3000
  Subtract : Sum
  Sum : Sum  Inputs=|+++-
  Sum1 : Sum  Inputs=|+-
  Sum2 : Sum  Inputs=|++-
  Switch Case Action Subsystem : Subsystem  TreatAsAtomicUnit=on
  Switch Case Action Subsystem1 : Subsystem  TreatAsAtomicUnit=on
  XF_XHZY : Saturate  UpperLimit=15  LowerLimit=-15
  XF_YJ : Saturate  UpperLimit=10  LowerLimit=-10
  ZXF_PID : Saturate  UpperLimit=2500  LowerLimit=-2500
  ZXF_PWM : Saturate  UpperLimit=4900  LowerLimit=100
  ZYDX_XHZY : Subsystem
  chu_jd : DataStoreRead  DataStoreName=chu_jd
  PWMOUT : Outport
  JD_Out : Outport  Port=2
  JD_Error : Outport  Port=3
  SGWY_Out : Outport  Port=4  OutDataTypeStr=int32
  wires:
  CDB_XHHY/1 -> Control_ZP/1(In_ZP)
  Control_ZP/1(Out_ZP) -> Saturation/1
  Sum1/1 -> Control_ZV/2(In_ZV)
  Control_ZV/1(Out_ZV) -> ZXF_PID/1
  ZXF_PID/1 -> Subtract/1
  Con_ZPWM/1 -> Subtract/2
  Subtract/1 -> ZXF_PWM/1
  ZXF_PWM/1 -> PWMOUT/1
  GXZ5/1 -> Sum1/2
  Encode_Sp/1 -> GXZ4/1
  GXZ4/1 -> GXZ5/1
  Encode_Pos/1 -> Data Type Conversion1/1
  ZYDX_XHZY/1(Zq) -> GXZ8/1
  GXZ7/1 -> KP_JD1/1, ZYDX_XHZY/1(Zl)
  GXZ8/1 -> Product3/2, KP_JD/1
  GXZ6/1 -> GXZ7/1, GXZ1/1
  GXZ3/1 -> GXZ10/1
  GXZ2/1 -> XF_YJ/1
  Saturation/1 -> Sum1/1, Saturation1/1
  GXZ1/1 -> GXZ9/1
  Product/1 -> Sum2/2
  XF_XHZY/1 -> Product1/2
  Product2/1 -> Sum/2
  KG_YJ/1 -> Product2/1
  KG_JD/1 -> Product1/1
  KG_En/1 -> Product/1
  Data Type Conversion1/1 -> GXZ6/1
  Data Type Conversion2/1 -> GXZ3/1
  Data Type Conversion3/1 -> GXZ2/1
  JD_In/1 -> If Action Subsystem3/1(In1), If Action Subsystem2/1(In1)
  If/1 -> If Action Subsystem3/Action
  If/2 -> If Action Subsystem1/Action
  If/3 -> If Action Subsystem2/Action
  Slect_port/1 -> If/1
  Data Store Read/1 -> Data Type Conversion2/1
  Data Store Read1/1 -> Data Type Conversion3/1
  YJ_In/1 -> If Action Subsystem3/2(In2), If Action Subsystem2/2(In2)
  Sum/1 -> JD_e(k)/1, KP_e/1
  GXZ9/1 -> Product/2
  KP_e/1 -> JD_Error/1
  KP_JD/1 -> JD_Out/1
  XF_YJ/1 -> Product2/2
  KP_JD1/1 -> Data Type Conversion4/1
  Data Type Conversion4/1 -> SGWY_Out/1
  GXZ10/1 -> XF_XHZY/1
  JD_e(k)/1 -> CDB_XHHY/1
  chu_jd/1 -> Sum/1
  Product3/1 -> Sum2/3
  EN_extern/1 -> Product3/1
  Sum2/1 -> Sum/4
  KG_JD1/1 -> If1/1
  If1/1 -> Switch Case Action Subsystem/Action
  Product1/1 -> Switch Case Action Subsystem1/1(In1), Switch Case Action Subsystem/1(In1)
  If1/2 -> Switch Case Action Subsystem1/Action
  Data Store Read2/1 -> Sum/3
  Data Store Read3/1 -> Sum2/1
  Forword/1 -> Product4/1
  Product4/1 -> Control_ZV/1(In_ZV1)
  Saturation1/1 -> Product4/2

== system motor/Chart/Open_Motor ==
  Encode_Sp : Inport  OutDataTypeStr=int32  PortDimensions=1
  f : TriggerPort  TriggerType=function-call
      settings: CopyFcn=Stateflow.SLINSF.SimulinkMan.removeBlockPreDeleteFcn  PreDeleteFcn=Stateflow.SLINSF.SimulinkMan.unsafePredeleteFcn
  Con_ZPWM : Constant  Value=2500
  GXZ4 : Gain  Gain=(360)/65536
  GXZ5 : Gain  Gain=500
  KG_clc : DataStoreRead  DataStoreName=KG_clc
  Product : Product
  SUDU_IN : Constant  Value=1200
  Subtract : Sum
  Sum1 : Sum  Inputs=|+-
  ZXF_PID : Saturate  UpperLimit=2500  LowerLimit=-2500
  ZXF_PWM : Saturate  UpperLimit=4800  LowerLimit=200
  sudu_PI : Subsystem
  PWMOUT : Outport
  wires:
  Sum1/1 -> sudu_PI/1(In_ZV)
  sudu_PI/1(Out_ZV) -> ZXF_PID/1
  ZXF_PID/1 -> Subtract/1
  Con_ZPWM/1 -> Subtract/2
  Subtract/1 -> ZXF_PWM/1
  ZXF_PWM/1 -> PWMOUT/1
  GXZ5/1 -> Sum1/2
  Encode_Sp/1 -> GXZ4/1
  GXZ4/1 -> GXZ5/1
  KG_clc/1 -> Product/1
  SUDU_IN/1 -> Product/2
  Product/1 -> Sum1/1

== system motor/Chart/Showing ==
  Showing_Angle : Inport
  Showing_T : Inport  Port=2
  f : TriggerPort  TriggerType=function-call
      settings: CopyFcn=Stateflow.SLINSF.SimulinkMan.removeBlockPreDeleteFcn  PreDeleteFcn=Stateflow.SLINSF.SimulinkMan.unsafePredeleteFcn
  Data Store Read : DataStoreRead  DataStoreName=Angle_S
  Data Store Write : DataStoreWrite  DataStoreName=Angle_S
  Data Type Conversion1 : DataTypeConversion  OutDataTypeStr=double
  Multiport Switch : MultiPortSwitch  Inputs=8
  Product : Product
  Sine Wave1 : Sin  Frequency=pi/3
  Sine Wave2 : Sin  Frequency=pi/4
  Sine Wave3 : Sin  Frequency=pi/5
  Sine Wave4 : Sin  Frequency=pi/6
  Sine Wave5 : Sin  Frequency=pi/8
  Sine Wave6 : Sin  Frequency=pi/10
  Sine Wave7 : Sin  Frequency=pi/13
  Sine Wave8 : Sin  Frequency=pi/15
  Angle : Outport
  wires:
  Showing_Angle/1 -> Product/2
  Product/1 -> Data Type Conversion1/1
  Data Store Read/1 -> Product/1
  Showing_T/1 -> Multiport Switch/1
  Multiport Switch/1 -> Data Store Write/1
  Sine Wave8/1 -> Multiport Switch/9
  Sine Wave7/1 -> Multiport Switch/8
  Sine Wave1/1 -> Multiport Switch/2
  Sine Wave2/1 -> Multiport Switch/3
  Sine Wave3/1 -> Multiport Switch/4
  Sine Wave4/1 -> Multiport Switch/5
  Sine Wave5/1 -> Multiport Switch/6
  Sine Wave6/1 -> Multiport Switch/7
  Data Type Conversion1/1 -> Angle/1

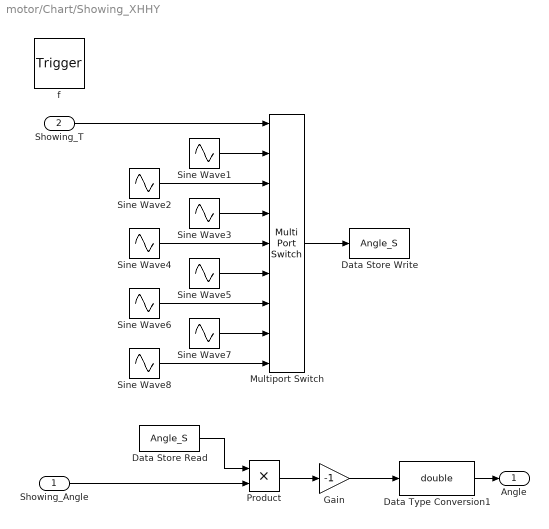
== system motor/Chart/Showing_XHHY ==
  Showing_Angle : Inport
  Showing_T : Inport  Port=2
  f : TriggerPort  TriggerType=function-call
      settings: CopyFcn=Stateflow.SLINSF.SimulinkMan.removeBlockPreDeleteFcn  PreDeleteFcn=Stateflow.SLINSF.SimulinkMan.unsafePredeleteFcn
  Data Store Read : DataStoreRead  DataStoreName=Angle_S
  Data Store Write : DataStoreWrite  DataStoreName=Angle_S
  Data Type Conversion1 : DataTypeConversion  OutDataTypeStr=double
  Gain : Gain  Gain=-1
  Multiport Switch : MultiPortSwitch  Inputs=8
  Product : Product
  Sine Wave1 : Sin  Frequency=pi/3  Phase=pi/2
  Sine Wave2 : Sin  Frequency=pi/4  Phase=pi/2
  Sine Wave3 : Sin  Frequency=pi/5  Phase=pi/2
  Sine Wave4 : Sin  Frequency=pi/6  Phase=pi/2
  Sine Wave5 : Sin  Frequency=pi/8  Phase=pi/2
  Sine Wave6 : Sin  Frequency=pi/10  Phase=pi/2
  Sine Wave7 : Sin  Frequency=pi/13  Phase=pi/2
  Sine Wave8 : Sin  Frequency=pi/15  Phase=pi/2
  Angle : Outport
  wires:
  Showing_Angle/1 -> Product/2
  Product/1 -> Gain/1
  Data Store Read/1 -> Product/1
  Showing_T/1 -> Multiport Switch/1
  Multiport Switch/1 -> Data Store Write/1
  Sine Wave8/1 -> Multiport Switch/9
  Sine Wave7/1 -> Multiport Switch/8
  Sine Wave1/1 -> Multiport Switch/2
  Sine Wave2/1 -> Multiport Switch/3
  Sine Wave3/1 -> Multiport Switch/4
  Sine Wave4/1 -> Multiport Switch/5
  Sine Wave5/1 -> Multiport Switch/6
  Sine Wave6/1 -> Multiport Switch/7
  Data Type Conversion1/1 -> Angle/1
  Gain/1 -> Data Type Conversion1/1

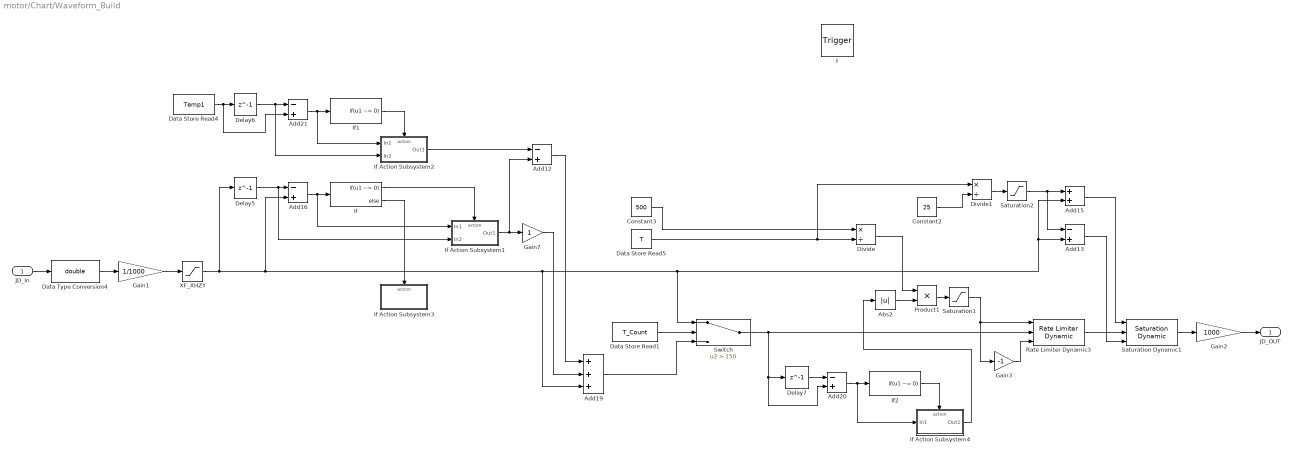
== system motor/Chart/Waveform_Build ==
  JD_In : Inport  OutDataTypeStr=int32  PortDimensions=1
  f : TriggerPort  TriggerType=function-call
      settings: CopyFcn=Stateflow.SLINSF.SimulinkMan.removeBlockPreDeleteFcn  PreDeleteFcn=Stateflow.SLINSF.SimulinkMan.unsafePredeleteFcn
  Abs2 : Abs
  Add{12..13,16,20..21} (5 alike) : Sum  Inputs=-+
  Add15 : Sum
  Add19 : Sum  Inputs=+++
  Constant2 : Constant  Value=25
  Constant3 : Constant  Value=500
  Data Store Read1 : DataStoreRead  DataStoreName=T_Count
  Data Store Read4 : DataStoreRead  DataStoreName=Temp1
  Data Store Read5 : DataStoreRead  DataStoreName=T
  Data Type Conversion4 : DataTypeConversion  OutDataTypeStr=double
  Delay5 : Delay  DelayLength=1
  Delay6 : Delay  DelayLength=1
  Delay7 : Delay  DelayLength=1
  Divide : Product  Inputs=*/
  Divide1 : Product  Inputs=*/
  Gain1 : Gain  Gain=1/1000
  Gain2 : Gain  Gain=1000  OutDataTypeStr=int32
  Gain3 : Gain  Gain=-1
  Gain7 : Gain
  If : If  IfExpression=u1 ~= 0
  If Action Subsystem1 : Subsystem  TreatAsAtomicUnit=on
  If Action Subsystem2 : Subsystem  TreatAsAtomicUnit=on
  If Action Subsystem3 : Subsystem  TreatAsAtomicUnit=on
  If Action Subsystem4 : Subsystem  TreatAsAtomicUnit=on
  If1 : If  IfExpression=u1 ~= 0  ShowElse=off
  If2 : If  IfExpression=u1 ~= 0  ShowElse=off
  Product1 : Product
  Rate Limiter Dynamic3 : simulink/Discontinuities/Rate Limiter Dynamic
  Saturation Dynamic1 : simulink/Discontinuities/Saturation Dynamic  OutMin=[]  OutMax=[]  OutDataTypeStr=Inherit: Same as second input  OutDataType=fixdt(1, 16)  OutScaling=2^-10  DoSatur=off
  Saturation1 : Saturate  UpperLimit=50  LowerLimit=0.01
  Saturation2 : Saturate  UpperLimit=5  LowerLimit=0.1
  Switch : Switch  Criteria=u2 > Threshold  Threshold=150
  XF_XHZY : Saturate  UpperLimit=25  LowerLimit=-25
  JD_OUT : Outport  OutDataTypeStr=int32
  wires:
  Gain3/1 -> Rate Limiter Dynamic3/3
  Abs2/1 -> Product1/2
  Add12/1 -> Add19/1
  Gain7/1 -> Add19/2
  Divide1/1 -> Saturation2/1
  If Action Subsystem4/1(Out1) -> Abs2/1
  Product1/1 -> Saturation1/1
  JD_In/1 -> Data Type Conversion4/1
  Saturation1/1 -> Rate Limiter Dynamic3/1, Gain3/1
  Rate Limiter Dynamic3/1 -> Saturation Dynamic1/2
  Saturation Dynamic1/1 -> Gain2/1
  Add15/1 -> Saturation Dynamic1/1
  Add13/1 -> Saturation Dynamic1/3
  Add16/1 -> If/1, If Action Subsystem1/1(In1)
  If/1 -> If Action Subsystem1/Action
  If Action Subsystem1/1(Out1) -> Add12/2, Gain7/1
  Delay5/1 -> If Action Subsystem1/2(In2), Add16/1
  Data Store Read4/1 -> Delay6/1, Add21/2
  Delay6/1 -> Add21/1, If Action Subsystem2/2(In2)
  Add21/1 -> If Action Subsystem2/1(In1), If1/1
  If1/1 -> If Action Subsystem2/Action
  If Action Subsystem2/1(Out1) -> Add12/1
  If/2 -> If Action Subsystem3/Action
  Data Store Read5/1 -> Divide1/1, Divide/2
  Constant3/1 -> Divide/1
  Divide/1 -> Product1/1
  Constant2/1 -> Divide1/2
  Switch/1 -> Delay7/1, Add20/2, Rate Limiter Dynamic3/2
  Delay7/1 -> Add20/1
  Add20/1 -> If2/1, If Action Subsystem4/1(In1)
  If2/1 -> If Action Subsystem4/Action
  Saturation2/1 -> Add15/1, Add13/1
  Data Store Read1/1 -> Switch/2
  Add19/1 -> Switch/3
  Gain1/1 -> XF_XHZY/1
  Data Type Conversion4/1 -> Gain1/1
  Gain2/1 -> JD_OUT/1
  XF_XHZY/1 -> Add15/2, Add13/2, Switch/1, Add19/3, Add16/2, Delay5/1

== system motor/Chart/Angle_Calculation/If Action Subsystem1 ==
  Encode_Pos : Inport  OutDataTypeStr=int32  PortDimensions=1
  Action Port : ActionPort  ActionType=elseif
  Data Type Conversion1 : DataTypeConversion  OutDataTypeStr=double
  GHDG5 : Gain  Gain=(-360)/65536
  GHDG7 : Gain  Gain=19*4/(360*39)
  GHDG8 : Gain  Gain=1/1000
  GHDG9 : Gain  Gain=(-180)/pi
  KP_JD : Gain  Gain=1000
  ZYDX_HYDG : Subsystem
  fk_dg3 : Gain
  JD_Out : Outport
  wires:
  Encode_Pos/1 -> Data Type Conversion1/1
  KP_JD/1 -> JD_Out/1
  Data Type Conversion1/1 -> GHDG5/1
  GHDG5/1 -> GHDG7/1
  GHDG7/1 -> GHDG8/1
  GHDG8/1 -> ZYDX_HYDG/1(l2)
  ZYDX_HYDG/1(x) -> GHDG9/1
  GHDG9/1 -> fk_dg3/1
  fk_dg3/1 -> KP_JD/1

== system motor/Chart/Angle_Calculation/If Action Subsystem2 ==
  Encode_Pos : Inport  OutDataTypeStr=int32  PortDimensions=1
  Action Port : ActionPort  ActionType=else
  Data Type Conversion1 : DataTypeConversion  OutDataTypeStr=double
  Data Type Conversion4 : DataTypeConversion  OutDataTypeStr=int32
  GXZ6 : Gain  Gain=(-360)/65536
  GXZ7 : Gain  Gain=19/(39*90)
  GXZ8 : Gain  Gain=(-180)/pi
  KP_JD : Gain  Gain=1000
  KP_JD1 : Gain  Gain=1000
  ZYDX_XHZY : Subsystem
  JD_Out : Outport
  SGWY_Out : Outport  Port=2  OutDataTypeStr=int32
  wires:
  Encode_Pos/1 -> Data Type Conversion1/1
  ZYDX_XHZY/1(Zq) -> GXZ8/1
  GXZ7/1 -> KP_JD1/1, ZYDX_XHZY/1(Zl)
  GXZ8/1 -> KP_JD/1
  GXZ6/1 -> GXZ7/1
  Data Type Conversion1/1 -> GXZ6/1
  KP_JD/1 -> JD_Out/1
  KP_JD1/1 -> Data Type Conversion4/1
  Data Type Conversion4/1 -> SGWY_Out/1

== system motor/Chart/Angle_Calculation/If Action Subsystem3 ==
  Encode_Pos : Inport  OutDataTypeStr=int32  PortDimensions=1
  SGWY_In : Inport  Port=2  OutDataTypeStr=int32  PortDimensions=1
  Action Port : ActionPort  ActionType=then
  Data Type Conversion1 : DataTypeConversion  OutDataTypeStr=double
  Data Type Conversion3 : DataTypeConversion  OutDataTypeStr=double
  GXH7 : Gain  Gain=(-180)/pi
  GXZ2 : Gain  Gain=1/1000
  GXZ6 : Gain  Gain=(-360)/65536
  GXZ7 : Gain  Gain=19/(39*90)
  KP_JD1 : Gain  Gain=1000
  ZYDX_XHHY : Subsystem
  JD_Out : Outport
  wires:
  Encode_Pos/1 -> Data Type Conversion1/1
  GXZ6/1 -> GXZ7/1
  Data Type Conversion1/1 -> GXZ6/1
  ZYDX_XHHY/1(Hq) -> GXH7/1
  GXZ7/1 -> ZYDX_XHHY/1(Hl)
  SGWY_In/1 -> Data Type Conversion3/1
  GXH7/1 -> KP_JD1/1
  GXZ2/1 -> ZYDX_XHHY/2(Zl)
  KP_JD1/1 -> JD_Out/1
  Data Type Conversion3/1 -> GXZ2/1

== system motor/Chart/Angle_Calculation_HY/fs_plat ==
  In1 : Inport
  GHDG7 : Gain  Gain=19*4/(360*39)
  GHDG8 : Gain  Gain=1/1000
  GHDG9 : Gain  Gain=(-180)/pi
  ZYDX_HYDG : Subsystem
  Out1 : Outport
  wires:
  GHDG7/1 -> GHDG8/1
  GHDG8/1 -> ZYDX_HYDG/1(l2)
  ZYDX_HYDG/1(x) -> GHDG9/1
  In1/1 -> GHDG7/1
  GHDG9/1 -> Out1/1

== system motor/Chart/BJ/If Action Subsystem ==
  In1 : Inport
  Action Port : ActionPort  ActionType=case
  If : If  IfExpression=u1 == 2  ElseIfExpressions=u1 == 3
  If Action Subsystem : Subsystem  TreatAsAtomicUnit=on
  If Action Subsystem1 : Subsystem  TreatAsAtomicUnit=on
  If Action Subsystem2 : Subsystem  TreatAsAtomicUnit=on
  wires:
  In1/1 -> If/1
  If/1 -> If Action Subsystem/Action
  If/3 -> If Action Subsystem2/Action
  If/2 -> If Action Subsystem1/Action

== system motor/Chart/BJ/If Action Subsystem1 ==
  In1 : Inport
  Action Port : ActionPort  ActionType=case
  If : If  IfExpression=u1 == 2  ElseIfExpressions=u1 == 3
  If Action Subsystem : Subsystem  TreatAsAtomicUnit=on
  If Action Subsystem1 : Subsystem  TreatAsAtomicUnit=on
  If Action Subsystem2 : Subsystem  TreatAsAtomicUnit=on
  wires:
  In1/1 -> If/1
  If/1 -> If Action Subsystem/Action
  If/3 -> If Action Subsystem2/Action
  If/2 -> If Action Subsystem1/Action

== system motor/Chart/BJ/If Action Subsystem2 ==
  In1 : Inport
  Action Port : ActionPort  ActionType=case
  If : If  IfExpression=u1 == 2  ElseIfExpressions=u1 == 3
  If Action Subsystem : Subsystem  TreatAsAtomicUnit=on
  If Action Subsystem1 : Subsystem  TreatAsAtomicUnit=on
  If Action Subsystem2 : Subsystem  TreatAsAtomicUnit=on
  wires:
  In1/1 -> If/1
  If/1 -> If Action Subsystem/Action
  If/3 -> If Action Subsystem2/Action
  If/2 -> If Action Subsystem1/Action

== system motor/Chart/Motor_HYDG/Control_ZP ==
  In_ZP : Inport
  Discrete-Time Integrator : DiscreteIntegrator  InitialConditionSetting=State (most efficient)  SampleTime=-1  ICPrevOutput=DiscIntNeverNeededParam  ICPrevScaledInput=DiscIntNeverNeededParam
  KD_KG : Gain  Gain=0
  Sum : Sum  Inputs=|+-
  Sum1 : Sum  Inputs=|++
  ZP_KN : Gain  Gain=100
  ZP_Kp : Gain  Gain=600
  ZP_Kp1 : Gain
  ZP_Kp2 : Gain  Gain=0.001
  ZV_KD1 : Gain  Gain=0.036
  Out_ZP : Outport
  wires:
  In_ZP/1 -> ZP_Kp/1
  ZP_Kp/1 -> ZP_Kp1/1, ZP_Kp2/1
  ZP_Kp2/1 -> ZV_KD1/1
  ZV_KD1/1 -> Sum/1
  Sum/1 -> ZP_KN/1
  Discrete-Time Integrator/1 -> Sum/2
  ZP_Kp1/1 -> Sum1/1
  Sum1/1 -> Out_ZP/1
  KD_KG/1 -> Sum1/2
  ZP_KN/1 -> Discrete-Time Integrator/1, KD_KG/1

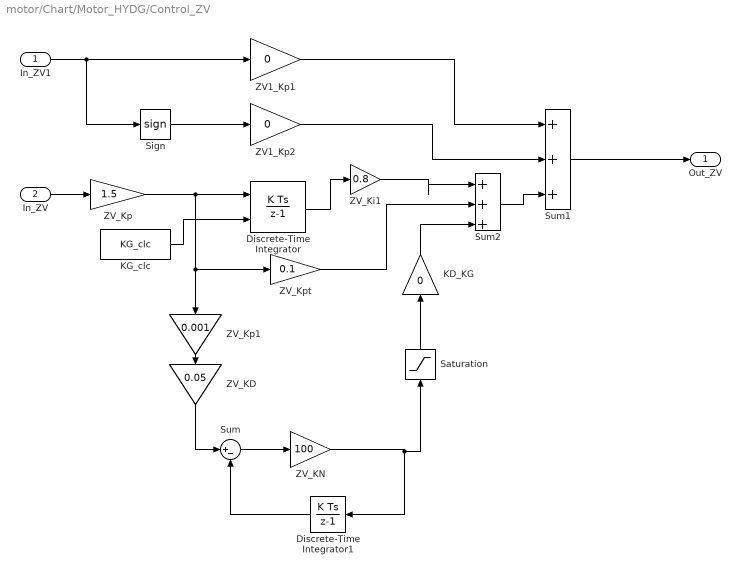
== system motor/Chart/Motor_HYDG/Control_ZV ==
  In_ZV1 : Inport
  In_ZV : Inport  Port=2
  Discrete-Time Integrator : DiscreteIntegrator  ExternalReset=either  SampleTime=-1  SaturateOnIntegerOverflow=on  LimitOutput=on  UpperSaturationLimit=2000  LowerSaturationLimit=-2000  ICPrevOutput=DiscIntNeverNeededParam  ICPrevScaledInput=DiscIntNeverNeededParam
  Discrete-Time Integrator1 : DiscreteIntegrator  InitialConditionSetting=State (most efficient)  SampleTime=-1  ICPrevOutput=DiscIntNeverNeededParam  ICPrevScaledInput=DiscIntNeverNeededParam
  KD_KG : Gain  Gain=0
  KG_clc : DataStoreRead  DataStoreName=KG_clc
  Saturation : Saturate  UpperLimit=300  LowerLimit=-300
  Sign : Signum
  Sum : Sum  Inputs=|+-
  Sum1 : Sum  Inputs=+++
  Sum2 : Sum  Inputs=|+++
  ZV1_Kp1 : Gain  Gain=0
  ZV1_Kp2 : Gain  Gain=0
  ZV_KD : Gain  Gain=0.05
  ZV_KN : Gain  Gain=100
  ZV_Ki1 : Gain  Gain=0.8
  ZV_Kp : Gain  Gain=1.5
  ZV_Kp1 : Gain  Gain=0.001
  ZV_Kpt : Gain  Gain=0.1
  Out_ZV : Outport
  wires:
  ZV_Kpt/1 -> Sum2/2
  Discrete-Time Integrator/1 -> ZV_Ki1/1
  In_ZV/1 -> ZV_Kp/1
  Sign/1 -> ZV1_Kp2/1
  In_ZV1/1 -> Sign/1, ZV1_Kp1/1
  Sum1/1 -> Out_ZV/1
  Sum2/1 -> Sum1/3
  ZV1_Kp2/1 -> Sum1/2
  ZV1_Kp1/1 -> Sum1/1
  ZV_Kp1/1 -> ZV_KD/1
  ZV_KD/1 -> Sum/1
  Sum/1 -> ZV_KN/1
  Discrete-Time Integrator1/1 -> Sum/2
  ZV_KN/1 -> Saturation/1, Discrete-Time Integrator1/1
  Saturation/1 -> KD_KG/1
  KD_KG/1 -> Sum2/3
  KG_clc/1 -> Discrete-Time Integrator/2
  ZV_Kp/1 -> Discrete-Time Integrator/1, ZV_Kp1/1, ZV_Kpt/1
  ZV_Ki1/1 -> Sum2/1

== system motor/Chart/Motor_HYDG/If Action Subsystem ==
  In1 : Inport
  Action Port : ActionPort  ActionType=then
  Data Store Write : DataStoreWrite  DataStoreName=JD_HYDG_HC
  Data Store Write1 : DataStoreWrite  DataStoreName=JD_HYDG
  wires:
  In1/1 -> Data Store Write1/1, Data Store Write/1

== system motor/Chart/Motor_HYDG/If Action Subsystem1 ==
  Action Port : ActionPort  ActionType=elseif
  Data Store Read : DataStoreRead  DataStoreName=JD_HYDG_HC
  Data Store Write1 : DataStoreWrite  DataStoreName=JD_HYDG
  wires:
  Data Store Read/1 -> Data Store Write1/1

== system motor/Chart/Motor_HYDG/If Action Subsystem2 ==
  In1 : Inport
  Action Port : ActionPort  ActionType=else
  Data Store Write : DataStoreWrite  DataStoreName=JD_HYDG_HC
  Data Store Write1 : DataStoreWrite  DataStoreName=JD_HYDG
  wires:
  In1/1 -> Data Store Write/1, Data Store Write1/1

== system motor/Chart/Motor_HYDG/fs_plat ==
  In1 : Inport
  GHDG7 : Gain  Gain=19*4/(360*39)
  GHDG8 : Gain  Gain=1/1000
  GHDG9 : Gain  Gain=(-180)/pi
  ZYDX_HYDG : Subsystem
  Out1 : Outport
  wires:
  GHDG7/1 -> GHDG8/1
  GHDG8/1 -> ZYDX_HYDG/1(l2)
  ZYDX_HYDG/1(x) -> GHDG9/1
  In1/1 -> GHDG7/1
  GHDG9/1 -> Out1/1

== system motor/Chart/Motor_HYDG1/Control_ZP ==
  In_ZP : Inport
  Discrete-Time Integrator : DiscreteIntegrator  InitialConditionSetting=State (most efficient)  SampleTime=-1  LimitOutput=on  UpperSaturationLimit=1000  LowerSaturationLimit=-1000  ICPrevOutput=DiscIntNeverNeededParam  ICPrevScaledInput=DiscIntNeverNeededParam
  KD_KG : Gain  Gain=100
  P_KP : DataStoreRead  DataStoreName=P_KP
  Product : Product
  Sum : Sum  Inputs=|+-
  Sum1 : Sum  Inputs=|++
  ZP_KN : Gain  Gain=400
  ZP_Kp : Gain
  ZV_KD1 : Gain  Gain=0.001
  Out_ZP : Outport
  wires:
  In_ZP/1 -> ZP_Kp/1
  ZV_KD1/1 -> Sum/1
  Sum/1 -> ZP_KN/1
  Discrete-Time Integrator/1 -> Sum/2
  Product/1 -> Sum1/1
  Sum1/1 -> Out_ZP/1
  KD_KG/1 -> Sum1/2
  ZP_KN/1 -> Discrete-Time Integrator/1, KD_KG/1
  ZP_Kp/1 -> ZV_KD1/1, Product/1
  P_KP/1 -> Product/2

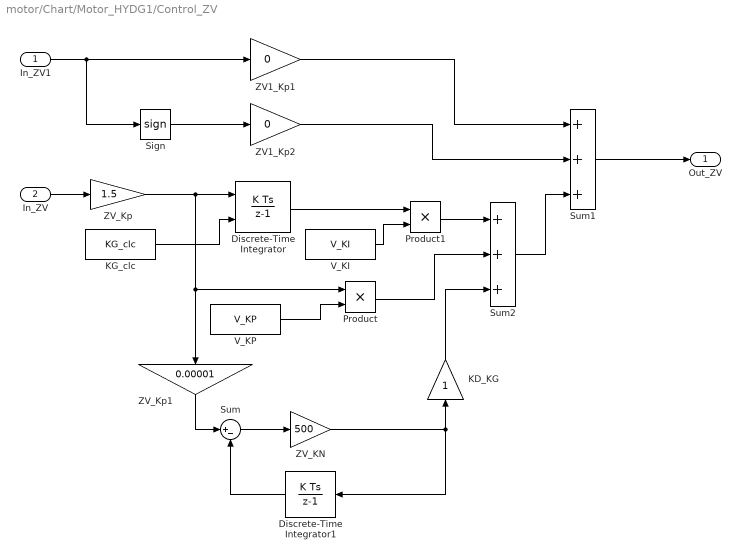
== system motor/Chart/Motor_HYDG1/Control_ZV ==
  In_ZV1 : Inport
  In_ZV : Inport  Port=2
  Discrete-Time Integrator : DiscreteIntegrator  ExternalReset=either  SampleTime=-1  SaturateOnIntegerOverflow=on  LimitOutput=on  UpperSaturationLimit=2000  LowerSaturationLimit=-2000  ICPrevOutput=DiscIntNeverNeededParam  ICPrevScaledInput=DiscIntNeverNeededParam
  Discrete-Time Integrator1 : DiscreteIntegrator  InitialConditionSetting=State (most efficient)  SampleTime=-1  LimitOutput=on  UpperSaturationLimit=1000  LowerSaturationLimit=-1000  ICPrevOutput=DiscIntNeverNeededParam  ICPrevScaledInput=DiscIntNeverNeededParam
  KD_KG : Gain
  KG_clc : DataStoreRead  DataStoreName=KG_clc
  Product : Product
  Product1 : Product
  Sign : Signum
  Sum : Sum  Inputs=|+-
  Sum1 : Sum  Inputs=+++
  Sum2 : Sum  Inputs=+++
  V_KI : DataStoreRead  DataStoreName=V_KI
  V_KP : DataStoreRead  DataStoreName=V_KP
  ZV1_Kp1 : Gain  Gain=0
  ZV1_Kp2 : Gain  Gain=0
  ZV_KN : Gain  Gain=500
  ZV_Kp : Gain  Gain=1.5
  ZV_Kp1 : Gain  Gain=0.00001
  Out_ZV : Outport
  wires:
  Product/1 -> Sum2/2
  Discrete-Time Integrator/1 -> Product1/1
  In_ZV/1 -> ZV_Kp/1
  Sign/1 -> ZV1_Kp2/1
  In_ZV1/1 -> Sign/1, ZV1_Kp1/1
  Sum1/1 -> Out_ZV/1
  Sum2/1 -> Sum1/3
  ZV1_Kp2/1 -> Sum1/2
  ZV1_Kp1/1 -> Sum1/1
  ZV_Kp1/1 -> Sum/1
  Sum/1 -> ZV_KN/1
  Discrete-Time Integrator1/1 -> Sum/2
  ZV_KN/1 -> KD_KG/1, Discrete-Time Integrator1/1
  KD_KG/1 -> Sum2/3
  KG_clc/1 -> Discrete-Time Integrator/2
  ZV_Kp/1 -> Discrete-Time Integrator/1, Product/1, ZV_Kp1/1
  Product1/1 -> Sum2/1
  V_KP/1 -> Product/2
  V_KI/1 -> Product1/2

== system motor/Chart/Motor_HYDG1/If Action Subsystem ==
  In1 : Inport
  Action Port : ActionPort  ActionType=then
  Data Store Write : DataStoreWrite  DataStoreName=JD_HYDG_HC
  Data Store Write1 : DataStoreWrite  DataStoreName=JD_HYDG
  wires:
  In1/1 -> Data Store Write1/1, Data Store Write/1

== system motor/Chart/Motor_HYDG1/If Action Subsystem1 ==
  Action Port : ActionPort  ActionType=elseif
  Data Store Read : DataStoreRead  DataStoreName=JD_HYDG_HC
  Data Store Write1 : DataStoreWrite  DataStoreName=JD_HYDG
  wires:
  Data Store Read/1 -> Data Store Write1/1

== system motor/Chart/Motor_HYDG1/If Action Subsystem2 ==
  In1 : Inport
  Action Port : ActionPort  ActionType=else
  Data Store Write : DataStoreWrite  DataStoreName=JD_HYDG_HC
  Data Store Write1 : DataStoreWrite  DataStoreName=JD_HYDG
  wires:
  In1/1 -> Data Store Write/1, Data Store Write1/1

== system motor/Chart/Motor_HYDG1/NYDX_HYDG ==
  qx : Inport
  Fcn : Fcn  Expr=0.1*(1-cos(u))
  Fcn1 : Fcn  Expr=u*u
  Fcn15 : Fcn  Expr=u-0.2655
  Fcn2 : Fcn  Expr=0.2655-0.1*sin(u)
  Fcn3 : Fcn  Expr=u*u
  Fcn4 : Fcn  Expr=sqrt(u)
  Sum1 : Sum  Inputs=|++
  l1 : Outport
  wires:
  Fcn15/1 -> l1/1
  Fcn4/1 -> Fcn15/1
  Sum1/1 -> Fcn4/1
  Fcn3/1 -> Sum1/2
  Fcn1/1 -> Sum1/1
  qx/1 -> Fcn2/1, Fcn/1
  Fcn2/1 -> Fcn3/1
  Fcn/1 -> Fcn1/1

== system motor/Chart/Motor_HYDG1/ZYDX_HYDG ==
  l2 : Inport
  Cl1 : Fcn  Expr=(2*0.1*0.1+0.2655*0.2655-u*u)/(2*0.1*0.1)
  Fcn : Fcn  Expr=(2.655-sqrt(2.655*2.655-u*u+1))/(u+1)
  Fcn4 : Fcn  Expr=2*atan(u)
  Fcn7 : Fcn  Expr=u+0.2655
  x : Outport
  wires:
  Fcn4/1 -> x/1
  l2/1 -> Fcn7/1
  Fcn/1 -> Fcn4/1
  Fcn7/1 -> Cl1/1
  Cl1/1 -> Fcn/1
